simulink model "mech_spen"  (Simulink 6.0)
settings: Solver=ode45  StartTime=0.0  StopTime=inf  RelTol=1e-5  AbsTol=1e-8
libraries: mblibv1 x5, simulink x1
settings Model: Creator=arnav  LastModifiedBy=batserve  ExtModeAutoUpdateStatusClock=off
settings DataIOCC: SignalLoggingName=sigsOut
settings OptimizationCC: BooleanDataType=off
settings DebuggingCC: CheckExecutionContextPreStartOutputMsg=on  CheckExecutionContextRuntimeOutputMsg=on  SolverPrmCheckMsg=none
settings HardwareCC: TargetUnknown=on

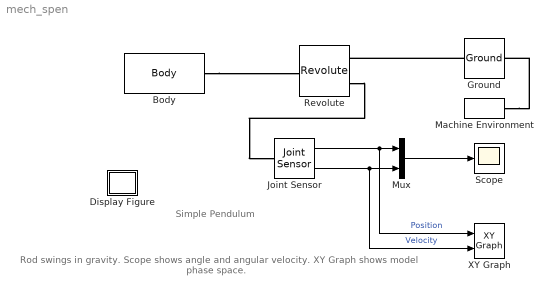
== system mech_spen ==
  note: Rod swings in gravity. Scope
      | shows angle and angular velocity.
      | XY Graph shows model phase space.
  note: Simple Pendulum
  Body : mblibv1/Bodies/Body  Orientation=left  PhysicalDomain=mechanical  SubClassName=Unknown  LeftPortType=workingframe  RightPortType=workingframe  LConnTagsString=CS1  DialogClass=MechanicalBodyBlock  Mass=2490  MassUnits=g  InertiaUnits=kg*m^2  Inertia=[ 1.25e-4 0 0; 0 0.208 0; 0 0 0.208]  Shape=Cylinder  ShapeDims=[1 1]  ShapeUnits=m  ShapeUse=false  Density=1  DensityUnits=kg/m^3  DensityUse=false  CG=Left$CG$[2.5 4 5]$WORLD$WORLD$m$[0 0 0]$Euler X-Y-Z$deg$WORLD$false  WorkingFrames=Left$CS1$[3 4 5]$WORLD$WORLD$m$[0 0 0]$Euler X-Y-Z$deg$WORLD$true
  Display Figure : Subsystem  Description="Help callback for simple pendulum model: mech_spen.mdl.  Opens Help browser to Type 19 marker at documentation for this tutorial model."
      settings: OpenFcn=pmhelpview([docroot '/toolbox/physmod/mech/mech.map'], 'mech_spen_help');
      mask Type: Help callback
      mask Display: image(imread('info.bmp'))
  Ground : mblibv1/Bodies/Ground  Orientation=left  Opaque=on  LeftPortType=env  RightPortType=workingframe  PhysicalDomain=Mechanical  DialogClass=GroundBlock  CoordPosition=[3 4 5]  CoordPositionUnits=m  StateVectorMgrId=-1  MachineId=[0 0]  ShowEnvPort=on
  Joint Sensor : mblibv1/Sensors &  Actuators/Joint Sensor  Opaque=on  PhysicalDomain=Mechanical  PortType=blob  Muxed=off  Pose=off  Angle=on  AngleUnits=deg  ArcVelocity=on  ArcVelocityUnits=deg/s  ArcAcceleration=off  ArcAccelerationUnits=deg/s^2  CoordPosition=on  CoordPositionUnits=m  Velocity=off  VelocityUnits=m/s  Acceleration=off  AccelerationUnits=m/s^2  Quaternion=on  QuaternionDT=off  QuaternionDDT=off  QuaternionUnits=off  OutputVector=[ 1 1 ]  ActiveIO=on  Width=2  DialogClass=MechanicalSensorBlock  Primitive=R1  Force=off  ForceUnits=N  Torque=off  TorqueUnits=N-m  ReferenceFrame=Absolute (INERTIAL)  ReactionSensedSide=Base  ReactionReferenceFrame=Absolute (World)  ReactionForce=off  ReactionForceUnits=N  ReactionMoment=off  ReactionMomentUnits=N-m
  Machine Environment : mblibv1/Bodies/Machine Environment  Tag=Factory ground  DialogController=MECH.DialogSource  Opaque=on  PortType=env  PhysicalDomain=Mechanical  DialogTemplateClass=MECH.MachineEnvironment  SyncWhenCopied=off  Gravity=[0 -9.81 0]  GravityUnits=m/s^2  GravityAsSignal=off  Dimensionality=3D Only  AnalysisType=Forward dynamics  LinearAssemblyTolerance=1e-3  LinearAssemblyToleranceUnits=m  AngularAssemblyTolerance=1e-3  AngularAssemblyToleranceUnits=rad  ConstraintSolverType=Stabilizing  ConstraintRelTolerance=1e-4  ConstraintAbsTolerance=1e-4  UseRobustSingularityHandling=off  StatePerturbationType=Fixed  PerturbationSize=1e-5  VisualizeMachine=on
  Mux : Mux  Inputs=2
  Revolute : mblibv1/Joints/Revolute  Orientation=left  PhysicalDomain=mechanical  SubClassName=Unknown  LeftPortType=blob  RightPortType=blob  LConnTagsString=__newl0|SA1  RConnTagsString=__newr0  NumSAPorts=1  CutJoint=off  MarkAsCut=off  Primitives=revolute  PrimitiveProps=R1$WORLD$[0 0 1]$revolute  DialogClass=JointBlock
  Scope : Scope
      settings: YMin=-350  YMax=350
  XY Graph : simulink/Sinks/XY Graph  xmin=-25  xmax=200  ymin=-500  ymax=500  st=-1
  wires:
  Joint Sensor/1 -> Mux/1, XY Graph/1  "Position"
  Joint Sensor/2 -> Mux/2, XY Graph/2  "Velocity"
  Mux/1 -> Scope/1
  connections:
  Ground/RConn1 -- Revolute/LConn1
  Revolute/LConn2 -- Joint Sensor/LConn1
  Body/LConn1 -- Revolute/RConn1
  Machine Environment/RConn1 -- Ground/LConn1

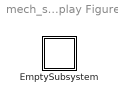
== system mech_spen/Display Figure ==
  EmptySubsystem : Subsystem

== system mech_spen/Display Figure/EmptySubsystem ==
